simulink model "DSLU_Model"  (R2016a)
settings: Solver=ode15s  StartTime=0.0  StopTime=195  RelTol=1e-4  AbsTol=1e-5
PreLoadFcn:
  | load UrbanCycle1
  | load UrbanCycle2
  | load UrbanCycle3
  | load UrbanCycle4
  | load UrbanCycle5
  | 
  | assignin('base','decimation',1)
  | Pbatt = 21e3;
  | Vbatt =100;
  | Ts = 6e-5;   % time step
  | 
  | Drive_Cycle_Num = 1;
  | warning off Simulink:Commands:LoadMdlParameterizedLink
  | 
  | HEV_Model_PARAM
PostLoadFcn:
  | warning off Simulink:Engine:UsingDefaultMaxStepSize
  | warning off Simulink:blocks:MatchingGotoNotFound
  | warning off Simulink:blocks:MatchingFromNotFound
  | warning off Simulink:blocks:TDelayBufferTooSmall
  | warning off Simulink:SL_SaveWithParameterizedLinks_Warning
  | warning off Simulink:SL_TDelayBufferTooSmall
  | warning off Simulink:SL_OutputNotConnected
  | warning off Simulink:SL_SaveWithDisabledLinks_Warning
  | 
  | warning off Simulink:SL_SetParamLinkChangeWarn
  | 
  | warning('off','Simulink:SL_UINotUpdatedDuringRapidAccelSim');
  | warning off Simulink:Engine:OutputNotConnected
  | warning off Simulink:Engine:UINotUpdatedDuringRapidAccelSim
  | warning off Simulink:Engine:SaveWithParameterizedLinks_Warning
  | warning off Simulink:Engine:SolverMaskedZC
  | set_param('HEV_SeriesParallel','MaskedZcDiagnostic','none');
  | warning off Simulink:Engine:SolverInconsistentInitialConditionsWarnForDAE
  | set_param('HEV_SeriesParallel','IgnoredZcDiagnostic','none');
  | warning off Simulink:Engine:SolverIgnoredZCBracketing
  | set_param('HEV_SeriesParallel','MaxConsecutiveZCsMsg','none');
  | warning off Simulink:Engine:SolverConsecutiveZCNum
  | warning off Simulink:Engine:SolverMinStepSizeWarnForDAE
  | warning off Simulink:Engine:SolverMinStepNonlinearIterWarnForDAE
  | warning off simscape:compiler:sli:init:SolverNotRecommended
  | warning off Simulink:Commands:SetParamLinkChangeWarn
  | warning off xPCTarget:sampleTime:sampleTimeInvariance
  | warning off Simulink:blocks:TDelayFixedBuffer
  | 
  | Setup_HEV_Model_Configurations
  | 
  | % Commands to avoid warning at first run
  | % PS battery function
  | warning off MATLAB:illConditionedMatrix
  | try
  |    set_param(bdroot, 'SimulationCommand', 'update');
  | catch
  | end
  | warning on MATLAB:illConditionedMatrix
model workspace (MAT data in the model file):
  guiH = 18054.0001221
undefined symbols (not defined in the file or in its folder): HEV_Param, sigbuilder_block
libraries: HEV_Electrical_Lib x6, HEV_Vehicle_Dynamics_Lib x2, fl_lib x1, slrtlib x1, nesl_utility x1, powerlib x1
Description:
  | Copyright 2014-2016 The MathWorks(TM), Inc.
settings Model: ExtModeTrigDuration=200  TunableVars=Drive_Cycle_Num  TunableVarsStorageClass=Auto  Creator=tegel  LastModifiedBy=ian.alferez
settings SolverCC: ZcThreshold=0  EnableConcurrentExecution=on  ZeroCrossAlgorithm=Adaptive
settings DataIOCC: SaveFormat=Array  SignalLoggingSaveFormat=ModelDataLogs  DSMLogging=off
settings OptimizationCC: BlockReduction=off  OptimizeBlockIOStorage=off  BufferReuse=off  GlobalBufferReuse=off  ExpressionFolding=off  ExpressionDepthLimit=2147483647  LocalBlockOutputs=off  InitFltsAndDblsToZero=on  EfficientMapNaN2IntZero=off
settings DebuggingCC: AlgebraicLoopMsg=error  UnderspecifiedInitializationDetection=Classic  MergeDetectMultiDrivingBlocksExec=none  SignalResolutionControl=TryResolveAllWithWarning  MaxConsecutiveZCsMsg=none  MaskedZcDiagnostic=none  IgnoredZcDiagnostic=none  MultiTaskDSMMsg=warning  MultiTaskCondExecSysMsg=none  SigSpecEnsureSampleTimeMsg=none  FcnCallInpInsideContextMsg=UseLocalSettings  AllowSymbolicDim=off  UnknownTsInhSupMsg=none  StateNameClashWarn=warning
settings HardwareCC: ProdBitPerPointer=32  ProdLargestAtomicFloat=None  ProdWordSize=32  ProdLongLongMode=on  ProdHWDeviceType=Generic->32-bit x86 compatible  TargetBitPerPointer=64  TargetLongLongMode=on  TargetIntDivRoundTo=Zero  TargetEndianess=LittleEndian  TargetWordSize=64  TargetHWDeviceType=MATLAB Host  ProdEqTarget=off
settings ModelReferenceCC: PropagateSignalLabelsOutOfModel=off
settings SFSimCC: SimParseCustomCode=off
settings RTWCC: Description=Generic Real-Time Target  RTWCompilerOptimization=on
settings GRTTargetCC: GeneratePreprocessorConditionals=Use local settings
settings ConfigComp: CovModelRefEnable=Off  CovSFcnEnable=off
settings SimscapeCC: ExplicitSolverDiagnosticOptions=none  SimscapeLogType=all  SimscapeLogName=simlog_HEVSP  SimscapeLogLimitData=off

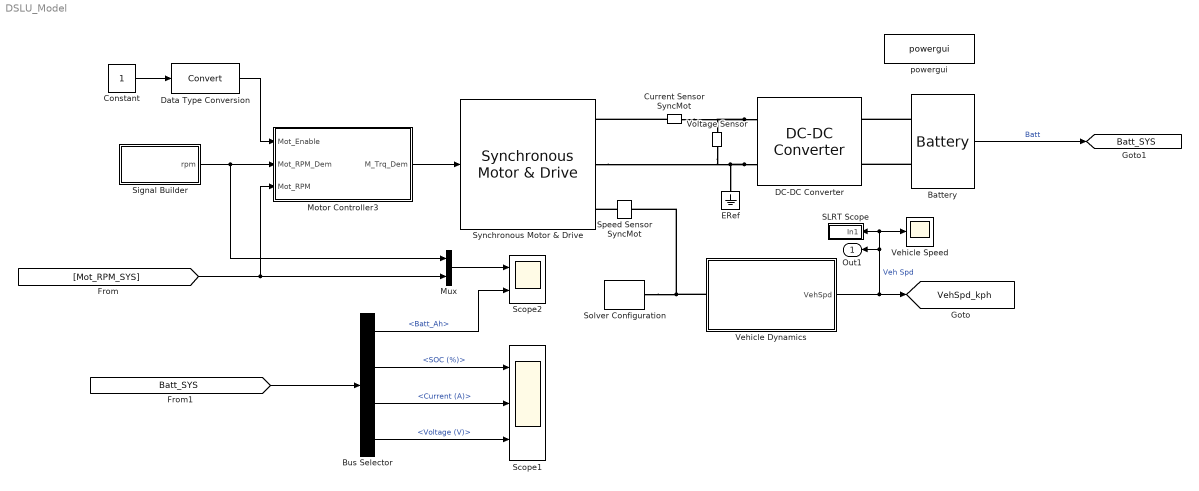
== system DSLU_Model ==
  Battery : HEV_Electrical_Lib/System Level/Battery  SystemSampleTime=-1  OverrideUsingVariant=Predefined
  Bus Selector : BusSelector  OutputSignals=Batt_Ah,SOC (%),Current (A),Voltage (V)
  Constant : Constant
  Current Sensor SyncMot : HEV_Electrical_Lib/System Level/Current Sensor SyncMot
  DC-DC Converter : HEV_Electrical_Lib/System Level/DC-DC Converter  Vout=HEV_Param.DCDCConv.Output_Voltage  RLoadLoss=HEV_Param.DCDCConv.Resistance_Losses  Kp=HEV_Param.DCDCConv.Kp  Ki=HEV_Param.DCDCConv.Ki
  Data Type Conversion : DataTypeConversion
  ERef : fl_lib/Electrical/Electrical Elements/Electrical Reference
  Motor Controller3 : Subsystem
  Mux : Mux  Inputs=2
  SLRT Scope : Subsystem
      mask Display: disp('SLRT')
  Scope1 : Scope  NumInputPorts=3
  Scope2 : Scope  NumInputPorts=2
  Signal Builder : Subsystem  Tag=STV Subsys  LoadFcn=sigbuilder_block('load');  StartFcn=sigbuilder_block('start');  StopFcn=sigbuilder_block('stop');  ClipboardFcn=sigbuilder_block('clipboard');  mask(Sigbuilder block){}
      mask help: Simulink:masks:SigbuilderBlock_MD
      mask init:
      | if ~strcmp(get_param(bdroot(gcbh),'SimulationStatus'),'stopped') tuvar = sigbuilder_block('maskInit'); end
      settings: CopyFcn=sigbuilder_block('copy');  DeleteFcn=sigbuilder_block('delete');  ModelCloseFcn=sigbuilder_block('modelClose');  PreSaveFcn=sigbuilder_block('preSave');  PauseFcn=sigbuilder_block('pause');  ContinueFcn=sigbuilder_block('continue');  NameChangeFcn=sigbuilder_block('namechange');  OpenFcn=sigbuilder_block('open',[275.5 73 550.5 362.5 ]);  CloseFcn=sigbuilder_block('close');
      mask Display: plot(0, 0, 100, 100,[2, 2, 32, 32, 2], [68, 8, 8, 68, 68],[32, 2], [38, 38], [32, 19, 2],[53, 60, 44], [32, 17, 17, 2],[16, 16, 31, 31]);txt = getActiveGroup(gcbh);text(2, 100, txt,'verticalAlignment', 'top');
  Solver Configuration : nesl_utility/Solver Configuration  PhysicalDomain=network_engine_domain  SubClassName=solver  LeftPortType=input  RightPortType=generic  Accelerate=off  Tones=[]  Harmonics=[]  SimulateNoise=off  Profile=off  UseLocalSampling=off  EnableSwitchedLinearOptims=on  FrequencyDomain=off  UseCCode=off  RelTol=0.001  AbsTol=1e-06  MinStep=1e-09  ToWorkspace=off  RevertToSquareIcSolve=off  NumHomotopyIterations=100  PhasorMode=off  PhasorModeNumHarmonics=1  OverrideAbsTol=off  DoDC=off  ResidualTolerance=1e-09  UseLocalSolver=off  LocalSolverChoice=NE_BACKWARD_EULER_ADVANCER  LocalSolverSampleTime=0.001  DoFixedCost=off  MaxNonlinIter=3  MaxModeIter=2  LinearAlgebra=Sparse  DelaysMemoryBudget=1024  AutomaticFiltering=on  FilteringTimeConstant=0.001
  Speed Sensor SyncMot : HEV_Electrical_Lib/System Level/Speed Sensor SyncMot  SystemSampleTime=-1
  Synchronous Motor & Drive : HEV_Electrical_Lib/System Level/Synchronous Motor & Drive  SystemSampleTime=-1
  Vehicle Speed : Scope
  Vehicle Dynamics : Subsystem  BlockChoice=Simple  Variant=on  OverrideUsingVariant=Full
      settings: AttributesFormatString=%<ActiveVariant>
      mask Display:
      | blk = find_system(gcbh, 'SearchDepth', 1, 'Parent', gcb, 'VariantObject', get_param(gcb,'activevariant'));
      | blk_mo = get_param(blk,'MaskObject');
      | iconCommands=blk_mo.Display;
      | commandCell=textscan(iconCommands,'%s','Delimiter','\n');
      | commandList=commandCell{:};
      | cellfun(@(x) eval(x), commandList);
  Voltage Sensor : HEV_Electrical_Lib/System Level/Voltage Sensor
  powergui : powerlib/powergui  SimulationMode=Continuous  SolverType=Tustin  SampleTime=Ts  frequency=60  SPID=on  DisableSnubberDevices=off  DisableRonSwitches=off  DisableVfSwitches=off  SwTol=0  DisplayEquations=off  Interpol=off  ExternalGateDelay=off  methode=off  Ts=0  FunctionMessages=off  echomessages=off  HookPort=off  EnableUseOfTLC=off  x0status=blocks  frequencyindice=0  Pbase=100e6  ErrMax=1e-4  Iterations=50  UnitsV=kV  UnitsW=MW  buscounter=0  RestoreLinks=warning  ResistiveCurrentMeasurement=off  Frange=[0:2:500]  Ylog=off  Xlog=on  ShowGrid=off  save=off  variable=ZData  structure=0  ZoomFFT=on  StartTime=0.0  cycles=1  DisplayStyle=1  fundamental=60  FreqAxis=off  MaxFrequency=1000  frequencyindicesteady=1  RmsSteady=1  display=off
  Out1 : Outport
  tag scope: Batt_SYS=global, VehSpd_kph=global
  wires:
  Vehicle Dynamics/1(VehSpd) -> [VehSpd_kph], Out1/1, SLRT Scope/1(In1), Vehicle Speed/1  "Veh Spd"
  Battery/1 -> [Batt_SYS]  "Batt"
  Motor Controller3/1(M_Trq_Dem) -> Synchronous Motor & Drive/1
  Data Type Conversion/1 -> Motor Controller3/1(Mot_Enable)
  Constant/1 -> Data Type Conversion/1
  Signal Builder/1(rpm) -> Mux/1, Motor Controller3/2(Mot_RPM_Dem)
  Mux/1 -> Scope2/1
  [Mot_RPM_SYS] -> Motor Controller3/3(Mot_RPM), Mux/2
  [Batt_SYS] -> Bus Selector/1
  Bus Selector/1 -> Scope2/2  "<Batt_Ah>"
  Bus Selector/2 -> Scope1/1  "<SOC (%)>"
  Bus Selector/3 -> Scope1/2  "<Current (A)>"
  Bus Selector/4 -> Scope1/3  "<Voltage (V)>"
  connections:
  Vehicle Dynamics/LConn1 -- Solver Configuration/RConn1 -- Speed Sensor SyncMot/RConn1
  DC-DC Converter/RConn2 -- ERef/LConn1 -- Voltage Sensor/RConn1 -- Synchronous Motor & Drive/RConn2
  DC-DC Converter/RConn1 -- Current Sensor SyncMot/LConn1 -- Voltage Sensor/LConn1
  Current Sensor SyncMot/RConn1 -- Synchronous Motor & Drive/RConn1
  Battery/LConn2 -- DC-DC Converter/LConn2
  Battery/LConn1 -- DC-DC Converter/LConn1
  Speed Sensor SyncMot/LConn1 -- Synchronous Motor & Drive/RConn3

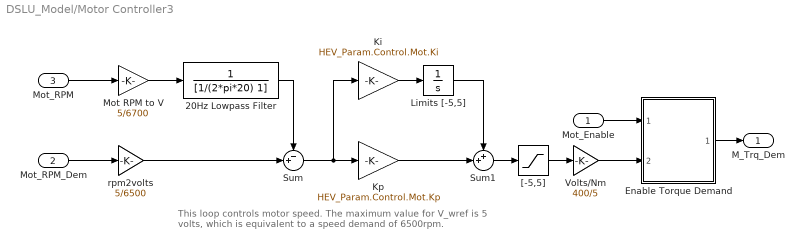
== system DSLU_Model/Motor Controller3 ==
  note: This loop controls motor speed. The maximum value
      | for V_wref is 5 volts, which is equivalent to a speed
      | demand of 6500rpm.
  Mot_Enable : Inport
  Mot_RPM_Dem : Inport  Port=2
  Mot_RPM : Inport  Port=3
  20Hz Lowpass Filter : TransferFcn  Denominator=[1/(2*pi*20) 1]
  Enable Torque Demand : Subsystem
  Ki : Gain  Gain=HEV_Param.Control.Mot.Ki
  Kp : Gain  Gain=HEV_Param.Control.Mot.Kp
  Limits [-5,5] : Integrator  LimitOutput=on  UpperSaturationLimit=5  LowerSaturationLimit=-5
  Mot RPM to V : Gain  Gain=5/6700
  Sum : Sum  Inputs=-+|
  Sum1 : Sum  Inputs=++|
  Volts/Nm : Gain  Gain=400/5
  "[-5,5]" : Saturate  UpperLimit=5  LowerLimit=-5
  rpm2volts : Gain  Gain=5/6500
  M_Trq_Dem : Outport
  wires:
  "[-5,5]"/1 -> Volts/Nm/1
  Mot_RPM/1 -> Mot RPM to V/1
  Sum1/1 -> "[-5,5]"/1
  Sum/1 -> Ki/1, Kp/1
  Ki/1 -> Limits [-5,5]/1
  Kp/1 -> Sum1/2
  Limits [-5,5]/1 -> Sum1/1
  20Hz Lowpass Filter/1 -> Sum/1
  rpm2volts/1 -> Sum/2
  Mot RPM to V/1 -> 20Hz Lowpass Filter/1
  Volts/Nm/1 -> Enable Torque Demand/2(TrqDemCtrl)
  Mot_RPM_Dem/1 -> rpm2volts/1
  Mot_Enable/1 -> Enable Torque Demand/1(Mot_Enable)
  Enable Torque Demand/1(TrqDem) -> M_Trq_Dem/1

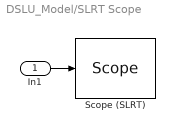
== system DSLU_Model/SLRT Scope ==
  In1 : Inport
  "Scope (SLRT) " : slrtlib/Displays and Logging/Scope   scopeno=1  scopetype=Target  autostart=on  viewmode=Graphical redraw  formatstr='%15.6f'  grid=on  ylimits=[-10,30]  nosamples=200  noprepostsamples=0  interleave=1  triggermode=FreeRun  triggersignal=1  trigsignalfromport=off  triggerlevel=0.0  triggerslope=Either  triggerscope=1  triggersample=0  filename=data.dat  mode=Lazy  writesize=512  autorestart=off  dynamicfilemode=off  maxwritefilesize=512*1024^2
  wires:
  In1/1 -> "Scope (SLRT) "/1

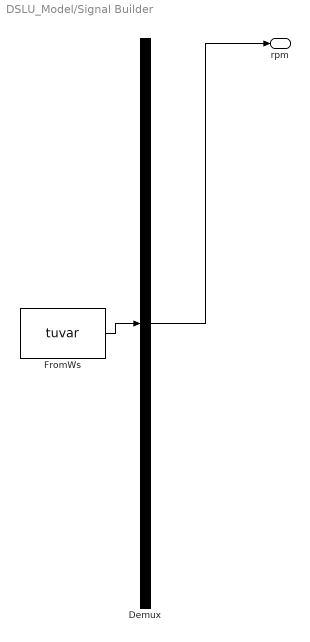
== system DSLU_Model/Signal Builder ==
  Demux : Demux  Tag=STV Demux  Outputs=1
  FromWs : FromWorkspace  Tag=STV FromWs  VariableName=tuvar  SampleTime=0
      SigBuilderData=|
      | common.afterFinalStr = 'Extrapolate'
      | common.sampleTime = 0
      | dataSet.timeRange = [0 195]
      | dataSet.name = 'Sheet1'
      | sbobj.Name = 'Signal Builder'
      | sbobj.Groups.Name = 'Sheet1'
      | sbobj.Groups.Signals.Name = 'rpm'
      | sbobj.Groups.Signals.XData = [0 1.01930209264e-06 1.01930209264e-06 1.02715101531e-06 1.03499993799e-06 1.04284886066e-06 1.12133808741e-06 1.19982731416e-06 1.27831654091e-06 1.54985777106e-06 1.82139900121e-06 2.09294023136e-06 ... (11789 elements, 1x11789)]
      | sbobj.Groups.Signals.YData = [0 0 0 0 0 0 0 0 0 0 0 0 ... (11789 elements, 1x11789)]
      | sbobj.Groups.TimeRange = [0 195]
  rpm : Outport
  wires:
  Demux/1 -> rpm/1
  FromWs/1 -> Demux/1

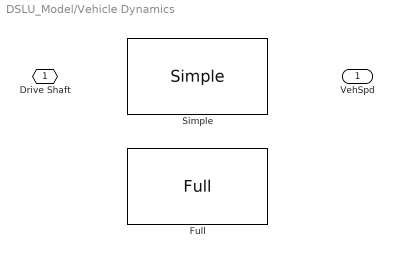
== system DSLU_Model/Vehicle Dynamics ==
  Full : HEV_Vehicle_Dynamics_Lib/Full  SystemSampleTime=-1  VariantControl=Full
  Simple : HEV_Vehicle_Dynamics_Lib/Simple  VariantControl=Simple  mass=HEV_Param.Vehicle.Mass  area=HEV_Param.Vehicle.Frontal_Area  Cd=HEV_Param.Vehicle.Aero_Drag_Coeff  radius=HEV_Param.Vehicle.Tire_Radius  wheel_inertia=HEV_Param.Vehicle.Wheel_Inertia  gear_ratio=HEV_Param.Vehicle.Engine_Vehicle_Gear_Ratio
  Drive Shaft : PMIOPort  Port=1  Side=Left
  VehSpd : Outport

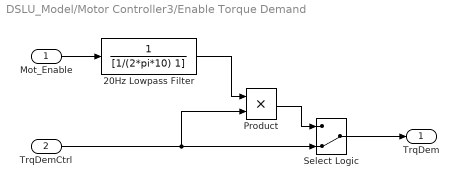
== system DSLU_Model/Motor Controller3/Enable Torque Demand ==
  Mot_Enable : Inport
  TrqDemCtrl : Inport  Port=2
  20Hz Lowpass Filter : TransferFcn  Denominator=[1/(2*pi*10) 1]
  Product : Product  RndMeth=Zero
  Select Logic : ManualSwitch  CurrentSetting=0
  TrqDem : Outport
  wires:
  Mot_Enable/1 -> 20Hz Lowpass Filter/1
  TrqDemCtrl/1 -> Product/2, Select Logic/2
  Product/1 -> Select Logic/1
  20Hz Lowpass Filter/1 -> Product/1
  Select Logic/1 -> TrqDem/1
